simulink model "SIL_PIL_torque"  (R2023b)
settings: Solver=FixedStepDiscrete  StartTime=0.0  StopTime=10.0  FixedStep=Ts  RelTol=1e-3  EnableMultiTasking=on
libraries: cstblocks x2
settings Model: ExtModeTrigDuration=10  Creator=giova  LastModifiedBy=giova
settings OptimizationCC: EnhancedBackFolding=on  PassReuseOutputArgsAs=Individual arguments  ZeroExternalMemoryAtStartup=off  ZeroInternalMemoryAtStartup=off  MaxStackSize=64  OptimizeBlockOrder=speed  DifferentSizesBufferReuse=on  OptimizationCustomize=off  EfficientTunableParamExpr=on
settings DebuggingCC: ParameterTunabilityLossMsg=error
settings HardwareCC: ProdBitPerPointer=32  ProdBitPerSizeT=32  ProdBitPerPtrDiffT=32  ProdLargestAtomicInteger=Long  ProdLargestAtomicFloat=Double  ProdWordSize=32  ProdLongLongMode=on  ProdHWDeviceType=ARM Compatible->ARM Cortex
settings SFSimCC: MATLABDynamicMemAlloc=off
settings RTWCC: Description=Embedded Coder  SystemTargetFile=ert.tlc  HardwareBoard=STM32 Nucleo F401RE  TemplateMakefile=ert_default_tmf  Toolchain=GNU Tools for ARM Embedded Processors  PortableWordSizes=on  CodeExecutionProfiling=on  CodeProfilingInstrumentation=coarse
settings CodeAppCC: ForceParamTrailComments=on  IgnoreCustomStorageClasses=off  OperatorAnnotations=on  SimulinkDataObjDesc=on  SFDataObjDesc=on  InsertBlockDesc=on
settings ERTTargetCC: ExtModeTransport=3  ExtModeStaticAlloc=on  ExtModeStaticAllocSize=2000  ExtModeMexFile=ext_xcp  ExtModeIntrfLevel=Level2 - Open

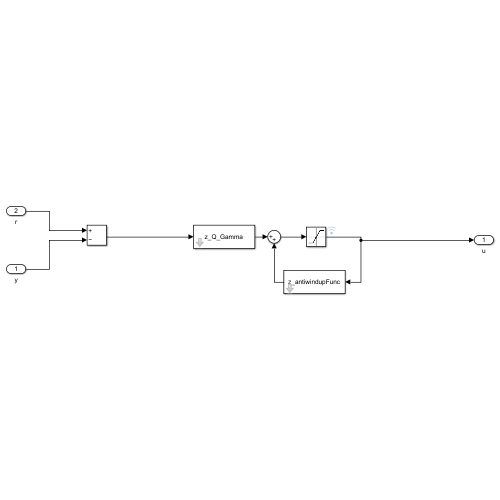
[thumbnail: Simulink's stored preview of the top-level diagram]
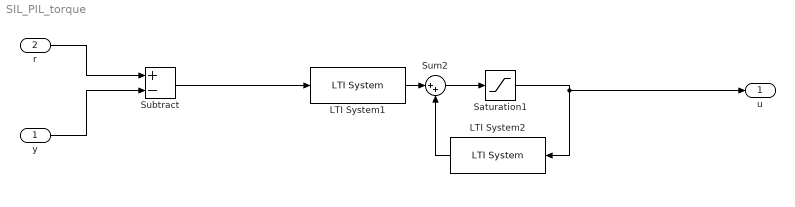
== system SIL_PIL_torque ==
  y : Inport
  r : Inport  Port=2
  LTI System1 : cstblocks/LTI System  sys=z_Q_Gamma  IC=[]  PadeOrder=0
  LTI System2 : cstblocks/LTI System  sys=z_antiwindupFunc  IC=[]  PadeOrder=0
  Saturation1 : Saturate  UpperLimit=12  LowerLimit=-12
  Subtract : Sum  Inputs=+-
  Sum2 : Sum  Inputs=|++
  u : Outport
  wires:
  Saturation1/1 -> u/1, LTI System2/1
  y/1 -> Subtract/2
  r/1 -> Subtract/1
  LTI System1/1 -> Sum2/1
  Subtract/1 -> LTI System1/1
  LTI System2/1 -> Sum2/2
  Sum2/1 -> Saturation1/1
